simulink model "simu_22a"  (R2022a)
settings: Solver=VariableStepAuto  StartTime=0.0  StopTime=5  RelTol=1e-3
settings Model: Creator=zhang  LastModifiedBy=psp_dada
settings ModelReferenceCC: EnableRefExpFcnMdlSchedulingChecks=off
settings RTWCC: Description=Generic Real-Time Target
settings ConfigComp: CovBoundaryAbsTol=1.0e-5

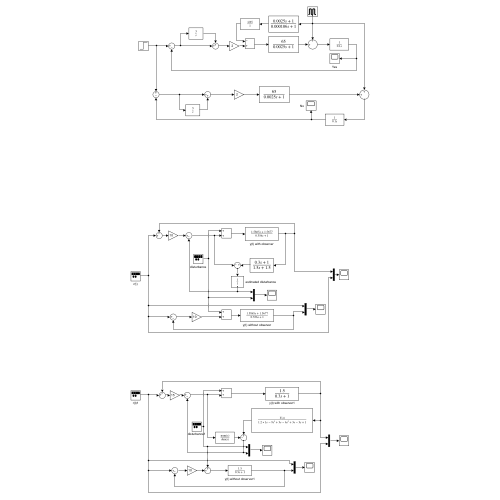
[thumbnail: Simulink's stored preview of the top-level diagram]
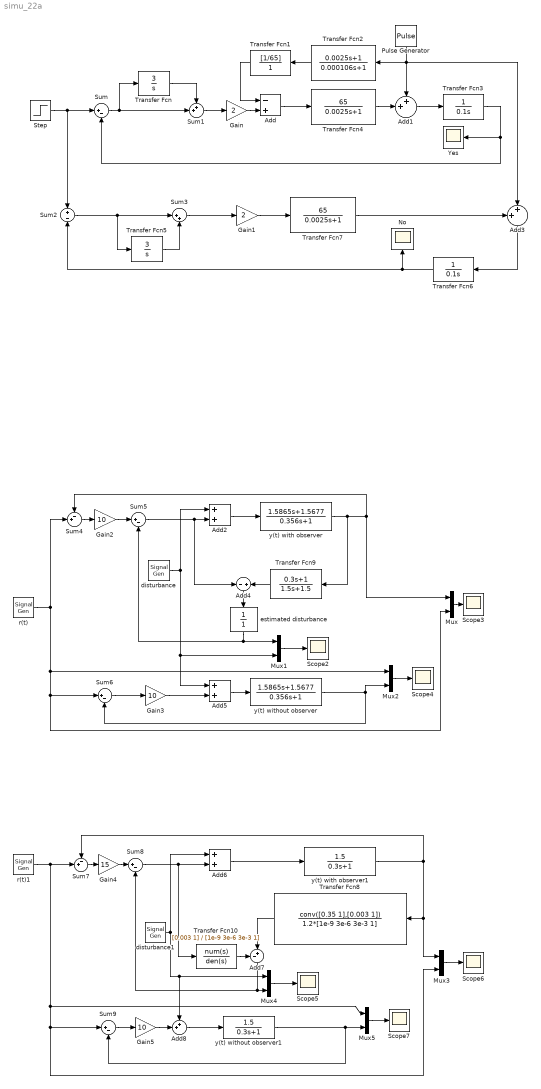
== system simu_22a ==
  Add : Sum  Inputs=-+
  Add1 : Sum  Inputs=++|
  Add2 : Sum
  Add3 : Sum  Inputs=++|
  Add4 : Sum  Inputs=-+
  Add5 : Sum
  Add6 : Sum
  Add7 : Sum  Inputs=-+|
  Add8 : Sum  Inputs=++|
  Gain : Gain  Gain=2
  Gain1 : Gain  Gain=2
  Gain2 : Gain  Gain=10
  Gain3 : Gain  Gain=10
  Gain4 : Gain  Gain=15
  Gain5 : Gain  Gain=10
  Mux{,1..5} (6 alike) : Mux  Inputs=2
  No : Scope
  Pulse Generator : DiscretePulseGenerator  PulseType=Time based  Amplitude=5  Period=0.2  PulseWidth=50
  Scope{2..7} (6 alike) : Scope
  Step : Step  SampleTime=0
  Sum{,5..6,8..9} (5 alike) : Sum  Inputs=|+-
  Sum1 : Sum  Inputs=++|
  Sum2 : Sum  Inputs=+|-
  Sum3 : Sum  Inputs=|++
  Sum4 : Sum  Inputs=-+|
  Sum7 : Sum  Inputs=-+|
  Transfer Fcn : TransferFcn  Numerator=[3]  Denominator=[1 0]
  Transfer Fcn1 : TransferFcn  Numerator=[1/65]  Denominator=[1]
  Transfer Fcn10 : TransferFcn  Numerator=[0.003 1]  Denominator=[1e-9 3e-6 3e-3 1]
  Transfer Fcn2 : TransferFcn  Numerator=[0.0025 1]  Denominator=[0.000106 1]
  Transfer Fcn3 : TransferFcn  Denominator=[0.1 0]
  Transfer Fcn4 : TransferFcn  Numerator=[65]  Denominator=[0.0025 1]
  Transfer Fcn5 : TransferFcn  Numerator=[3]  Denominator=[1 0]
  Transfer Fcn6 : TransferFcn  Denominator=[0.1 0]
  Transfer Fcn7 : TransferFcn  Numerator=[65]  Denominator=[0.0025 1]
  Transfer Fcn8 : TransferFcn  Numerator=conv([0.35 1],[0.003 1])  Denominator=1.2*[1e-9 3e-6 3e-3 1]
  Transfer Fcn9 : TransferFcn  Numerator=[0.3 1]  Denominator=[1.5 1.5]
  Yes : Scope
  disturbance : SignalGenerator  Amplitude=5  Frequency=200
  disturbance1 : SignalGenerator  Amplitude=5  Frequency=26
  estimated disturbance : TransferFcn  Denominator=[1]
  r(t) : SignalGenerator  Frequency=2
  r(t)1 : SignalGenerator  Frequency=2
  y(t) with observer : TransferFcn  Numerator=[1.5865 1.5677]  Denominator=[0.356 1]
  y(t) with observer1 : TransferFcn  Numerator=[1.5]  Denominator=[0.3 1]
  y(t) without observer : TransferFcn  Numerator=[1.5865 1.5677]  Denominator=[0.356 1]
  y(t) without observer1 : TransferFcn  Numerator=[1.5]  Denominator=[0.3 1]
  wires:
  Transfer Fcn3/1 -> Sum/2, Yes/1
  Sum/1 -> Sum1/2, Transfer Fcn/1
  Transfer Fcn/1 -> Sum1/1
  Sum1/1 -> Gain/1
  Gain/1 -> Add/2
  Transfer Fcn1/1 -> Add/1
  Transfer Fcn2/1 -> Transfer Fcn1/1
  Add/1 -> Transfer Fcn4/1
  Transfer Fcn4/1 -> Add1/2
  Sum3/1 -> Gain1/1
  Step/1 -> Sum2/1, Sum/1
  Sum2/1 -> Transfer Fcn5/1, Sum3/1
  Transfer Fcn6/1 -> Sum2/2, No/1
  Gain1/1 -> Transfer Fcn7/1
  Add3/1 -> Transfer Fcn6/1
  Transfer Fcn7/1 -> Add3/1
  Transfer Fcn5/1 -> Sum3/2
  Pulse Generator/1 -> Add1/1, Add3/2, Transfer Fcn2/1
  Sum5/1 -> Add4/1, Add2/2
  Transfer Fcn9/1 -> Add4/2
  Add4/1 -> estimated disturbance/1
  estimated disturbance/1 -> Sum5/2, Mux1/1
  Gain2/1 -> Sum5/1
  Add2/1 -> y(t) with observer/1
  y(t) with observer/1 -> Sum4/1, Mux/1, Transfer Fcn9/1
  Sum4/1 -> Gain2/1
  r(t)/1 -> Sum4/2, Mux/2, Sum6/1, Mux2/1
  disturbance/1 -> Add2/1, Mux1/2, Add5/1
  Mux1/1 -> Scope2/1
  Mux/1 -> Scope3/1
  Gain3/1 -> Add5/2
  Add5/1 -> y(t) without observer/1
  Sum6/1 -> Gain3/1
  Mux2/1 -> Scope4/1
  y(t) without observer/1 -> Mux2/2, Sum6/2
  Gain5/1 -> Add8/2
  Sum7/1 -> Gain4/1
  Add7/1 -> Sum8/2, Mux4/2
  y(t) without observer1/1 -> Sum9/2, Mux5/2
  Mux4/1 -> Scope5/1
  disturbance1/1 -> Add6/1, Mux4/1, Add8/1
  Sum9/1 -> Gain5/1
  y(t) with observer1/1 -> Mux3/1, Transfer Fcn8/1, Sum7/1
  r(t)1/1 -> Mux3/2, Sum9/1, Mux5/1, Sum7/2
  Gain4/1 -> Sum8/1
  Sum8/1 -> Transfer Fcn10/1, Add6/2
  Mux5/1 -> Scope7/1
  Add6/1 -> y(t) with observer1/1
  Add8/1 -> y(t) without observer1/1
  Transfer Fcn8/1 -> Add7/2
  Mux3/1 -> Scope6/1
  Transfer Fcn10/1 -> Add7/1
  Add1/1 -> Transfer Fcn3/1
